simulink model "Faultanalysis3phase"  (Simulink 9.3)
settings: Solver=ode45  StartTime=0.0  StopTime=0.5  RelTol=1e-3  EnableMultiTasking=on
libraries: powerlib x11, simulink_extras x3
settings Model: Creator=Administrator  LastModifiedBy=Psyna
settings DataIOCC: LimitDataPoints=on
settings OptimizationCC: ExpressionDepthLimit=2147483647
settings DebuggingCC: SolverPrmCheckMsg=warning  StateNameClashWarn=warning
settings GRTTargetCC: GeneratePreprocessorConditionals=Disable all
settings ConfigComp: CovSFcnEnable=off
settings SimscapeCC: SimscapeNormalizeSystem=off

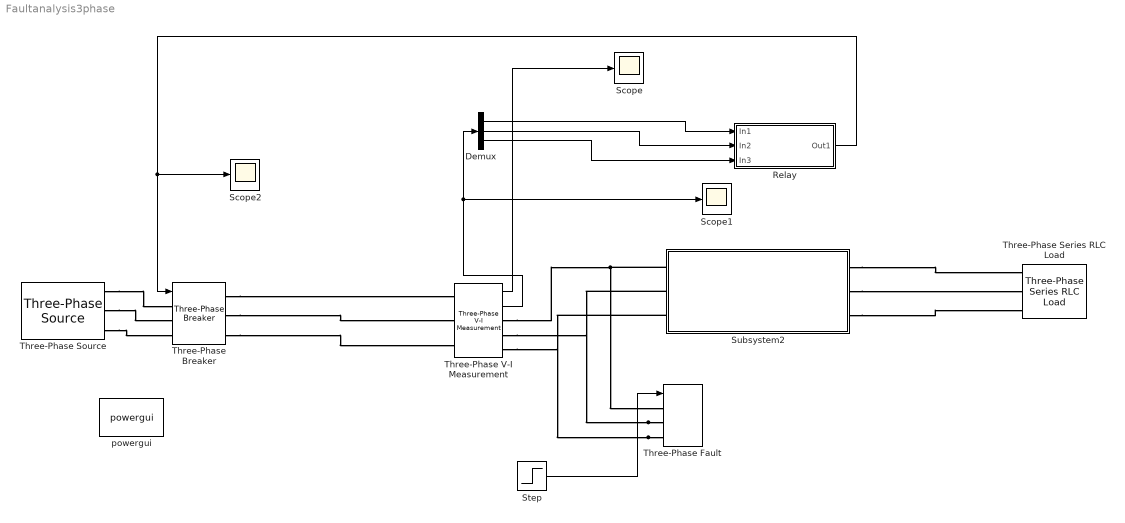
== system Faultanalysis3phase ==
  Demux : Demux  Outputs=3
  "Relay " : Subsystem
  Scope : Scope
  Scope1 : Scope
  Scope2 : Scope
  Step : Step  Time=0.15  SampleTime=0
  Subsystem2 : Subsystem
  Three-Phase Series RLC Load : powerlib/Elements/Three-Phase Series RLC Load  LConnTagsString=A|B|C  Configuration=Y (grounded)  NominalVoltage=500e3  Vabc=[1e3 1e3 1e3]  Vabcp=[1e3 1e3 1e3]  NominalFrequency=50  UnbalancedPower=off  ActivePower=200e6  InductivePower=100  CapacitivePower=0  Pabc=[10e3 9e3 11e3]  QLabc=[100 90 110]  QCabc=[100 90 110]  Pabcp=[10e3 9e3 11e3]  QLabcp=[100 90 110]  QCabcp=[100 90 110]  Measurements=None  LoadType=constant Z
      settings: SourceProductName=Simscape Electrical
  Three-Phase V-I Measurement : powerlib/Measurements/Three-Phase V-I Measurement  VoltageMeasurement=phase-to-ground  SetLabelV=off  LabelV=Vabc  Vpu=off  VpuLL=off  CurrentMeasurement=yes  SetLabelI=off  LabelI=Iabc  Ipu=off  Pbase=100e6  Vbase=11e3  OutputType=Complex  PhasorSimulation=off  PSBequivalent=0
      settings: SourceProductName=Simscape Electrical
  Three-Phase Breaker : powerlib/Elements/Three-Phase Breaker  InitialState=closed  SwitchA=on  SwitchB=on  SwitchC=on  SwitchTimes="[4/60  10/60]"  External=on  BreakerResistance=0.001  SnubberResistance=1e6  SnubberCapacitance=inf  Measurements=None
      settings: SourceProductName=Simscape Electrical
  Three-Phase Fault : powerlib/Elements/Three-Phase Fault  InitialStates=0  FaultA=on  FaultB=on  FaultC=on  GroundFault=on  SwitchTimes=[ 0.1 0.2]  External=on  SwitchStatus=NaN  FaultResistance=0.001  GroundResistance=0.001  SnubberResistance=1e6  SnubberCapacitance=inf  Measurements=None
      settings: SourceProductName=Simscape Electrical
  Three-Phase Source : powerlib/Electrical Sources/Three-Phase Source  InternalConnection=Yg  VoltagePhases=off  Voltage=500e3  PhaseAngle=0  Voltage_phases=[25e3 25e3 25e3]/sqrt(3)  PhaseAngles_phases=[0 -120 +120]  Frequency=50  NonIdealSource=on  SpecifyImpedance=on  Resistance=0.8929  Inductance=16.58e-3  ShortCircuitLevel=500e12  BaseVoltage=500e3  XRratio=7  BusType=swing  Pref=0  Qref=0  Prefabc=[10e3, 10e3, 10e3]  Qrefabc=[0, 0, 0]  Qmin=-inf  Qmax=inf
      settings: SourceProductName=Simscape Electrical
  powergui : powerlib/powergui  Priority=1  SimulationMode=Discrete  SampleTime=1e-4  frequency=60  Iterations=50  frequencyindice=50  Pbase=100e6  ErrMax=1e-4  UnitsV=kV  UnitsW=MW  buscounter=0  FunctionMessages=off  echomessages=off  EnableUseOfTLC=off  CurrentSourceSwitches=off  DisableSnubberDevices=off  DisableRonSwitches=off  DisableVfSwitches=off  DisplayEquations=off  AutomaticDiscreteSolvers=off  SolverType=Tustin  Interpol=off  ExternalGateDelay=off  methode=off  Ts=0  x0status=blocks  SPID=off  SwTol=0  HookPort=off  NonlinearTolerance=0  nMaxIteration=15  ContinueOnMaxIteration=off  RestoreLinks=warning  ResistiveCurrentMeasurement=off  Frange=[0:2:500]  Ylog=off  Xlog=on  ShowGrid=off  save=off  variable=ZData  structure=0  ZoomFFT=off  StartTime=0.0  cycles=1  DisplayStyle=1  fundamental=60  FreqAxis=off  MaxFrequency=1000  frequencyindicesteady=1  RmsSteady=1  display=off
      settings: SourceProductName=Simscape Electrical
  wires:
  Three-Phase V-I Measurement/2 -> Scope1/1, Demux/1
  Demux/1 -> "Relay "/1(In1)
  Demux/2 -> "Relay "/2(In2)
  Demux/3 -> "Relay "/3(In3)
  Three-Phase V-I Measurement/1 -> Scope/1
  Step/1 -> Three-Phase Fault/1
  "Relay "/1(Out1) -> Three-Phase Breaker/1, Scope2/1
  connections:
  Three-Phase Source/RConn3 -- Three-Phase Breaker/LConn3
  Three-Phase Source/RConn2 -- Three-Phase Breaker/LConn2
  Three-Phase Source/RConn1 -- Three-Phase Breaker/LConn1
  Three-Phase V-I Measurement/RConn1 -- Three-Phase Fault/LConn1 -- Subsystem2/LConn1
  Three-Phase Fault/LConn3 -- Subsystem2/LConn3 -- Three-Phase V-I Measurement/RConn3
  Subsystem2/RConn3 -- Three-Phase Series RLC Load/LConn3
  Subsystem2/RConn2 -- Three-Phase Series RLC Load/LConn2
  Subsystem2/RConn1 -- Three-Phase Series RLC Load/LConn1
  Three-Phase Fault/LConn2 -- Subsystem2/LConn2 -- Three-Phase V-I Measurement/RConn2
  Three-Phase Breaker/RConn1 -- Three-Phase V-I Measurement/LConn1
  Three-Phase Breaker/RConn2 -- Three-Phase V-I Measurement/LConn2
  Three-Phase Breaker/RConn3 -- Three-Phase V-I Measurement/LConn3

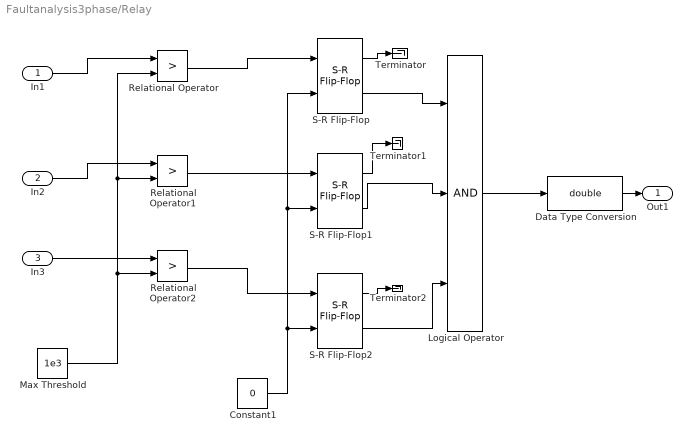
== system Faultanalysis3phase/Relay  ==
  In1 : Inport
  In2 : Inport  Port=2
  In3 : Inport  Port=3
  Constant1 : Constant  Value=0  OutDataTypeStr=boolean
  Data Type Conversion : DataTypeConversion  OutDataTypeStr=double
  Logical Operator : Logic  Inputs=3  AllPortsSameDT=off  OutDataTypeStr=boolean
  "Max Threshold " : Constant  Value=1e3
  Relational Operator : RelationalOperator  Operator=>  OutDataTypeStr=boolean  RndMeth=Nearest
  Relational Operator1 : RelationalOperator  Operator=>  OutDataTypeStr=boolean  RndMeth=Nearest
  Relational Operator2 : RelationalOperator  Operator=>  OutDataTypeStr=boolean  RndMeth=Nearest
  S-R Flip-Flop : simulink_extras/Flip Flops/S-R Flip-Flop  initial_condition=0
  S-R Flip-Flop1 : simulink_extras/Flip Flops/S-R Flip-Flop  initial_condition=0
  S-R Flip-Flop2 : simulink_extras/Flip Flops/S-R Flip-Flop  initial_condition=0
  Terminator : Terminator
  Terminator1 : Terminator
  Terminator2 : Terminator
  Out1 : Outport
  wires:
  In1/1 -> Relational Operator/1
  In2/1 -> Relational Operator1/1
  In3/1 -> Relational Operator2/1
  "Max Threshold "/1 -> Relational Operator/2, Relational Operator1/2, Relational Operator2/2
  Relational Operator/1 -> S-R Flip-Flop/1
  Relational Operator1/1 -> S-R Flip-Flop1/1
  Relational Operator2/1 -> S-R Flip-Flop2/1
  Constant1/1 -> S-R Flip-Flop2/2, S-R Flip-Flop/2, S-R Flip-Flop1/2
  S-R Flip-Flop/2 -> Logical Operator/1
  S-R Flip-Flop1/2 -> Logical Operator/2
  S-R Flip-Flop2/2 -> Logical Operator/3
  S-R Flip-Flop2/1 -> Terminator2/1
  S-R Flip-Flop1/1 -> Terminator1/1
  S-R Flip-Flop/1 -> Terminator/1
  Logical Operator/1 -> Data Type Conversion/1
  Data Type Conversion/1 -> Out1/1

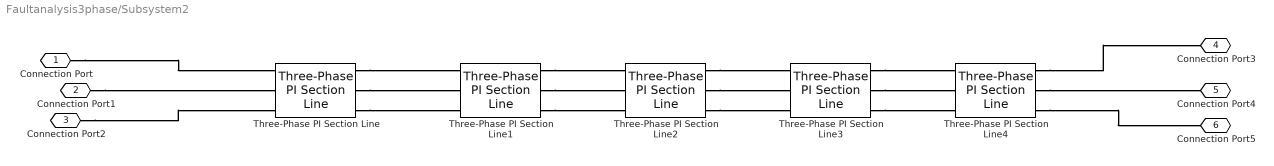
== system Faultanalysis3phase/Subsystem2 ==
  Three-Phase PI Section Line{,1..4} (5 alike) : powerlib/Elements/Three-Phase PI Section Line  LConnTagsString=a|b|c  RConnTagsString=A|B|C  Frequency=50  Resistances=[ 0.01273 0.3864]  Inductances="[ 0.9337e-3  4.1264e-3]"  Capacitances=[12.74e-9 7.751e-9]  Length=30
      settings: SourceProductName=Simscape Electrical
  Connection Port : PMIOPort  Side=Left
  Connection Port1 : PMIOPort  Port=2  Side=Left
  Connection Port2 : PMIOPort  Port=3  Side=Left
  Connection Port3 : PMIOPort  Port=4  Side=Right
  Connection Port4 : PMIOPort  Port=5  Side=Right
  Connection Port5 : PMIOPort  Port=6  Side=Right
  connections:
  Three-Phase PI Section Line4/RConn2 -- Connection Port4/RConn1
  Three-Phase PI Section Line1/RConn2 -- Three-Phase PI Section Line2/LConn2
  Three-Phase PI Section Line/RConn2 -- Three-Phase PI Section Line1/LConn2
  Connection Port2/RConn1 -- Three-Phase PI Section Line/LConn3
  Three-Phase PI Section Line2/RConn2 -- Three-Phase PI Section Line3/LConn2
  Three-Phase PI Section Line3/RConn2 -- Three-Phase PI Section Line4/LConn2
  Three-Phase PI Section Line/RConn1 -- Three-Phase PI Section Line1/LConn1
  Three-Phase PI Section Line3/RConn1 -- Three-Phase PI Section Line4/LConn1
  Three-Phase PI Section Line4/RConn1 -- Connection Port3/RConn1
  Three-Phase PI Section Line1/RConn1 -- Three-Phase PI Section Line2/LConn1
  Three-Phase PI Section Line3/RConn3 -- Three-Phase PI Section Line4/LConn3
  Three-Phase PI Section Line4/RConn3 -- Connection Port5/RConn1
  Three-Phase PI Section Line1/RConn3 -- Three-Phase PI Section Line2/LConn3
  Connection Port/RConn1 -- Three-Phase PI Section Line/LConn1
  Connection Port1/RConn1 -- Three-Phase PI Section Line/LConn2
  Three-Phase PI Section Line/RConn3 -- Three-Phase PI Section Line1/LConn3
  Three-Phase PI Section Line2/RConn3 -- Three-Phase PI Section Line3/LConn3
  Three-Phase PI Section Line2/RConn1 -- Three-Phase PI Section Line3/LConn1
